simulink subsystem "HO_VectorBox"  (R2019b)
settings: Solver=VariableStepAuto  StartTime=0.0  StopTime=10.0  RelTol=1e-3
libraries: canmsglib x8, c280xlib x8, FunctionCallDivider x3
settings Model: Creator=Nick  LastModifiedBy=Nick

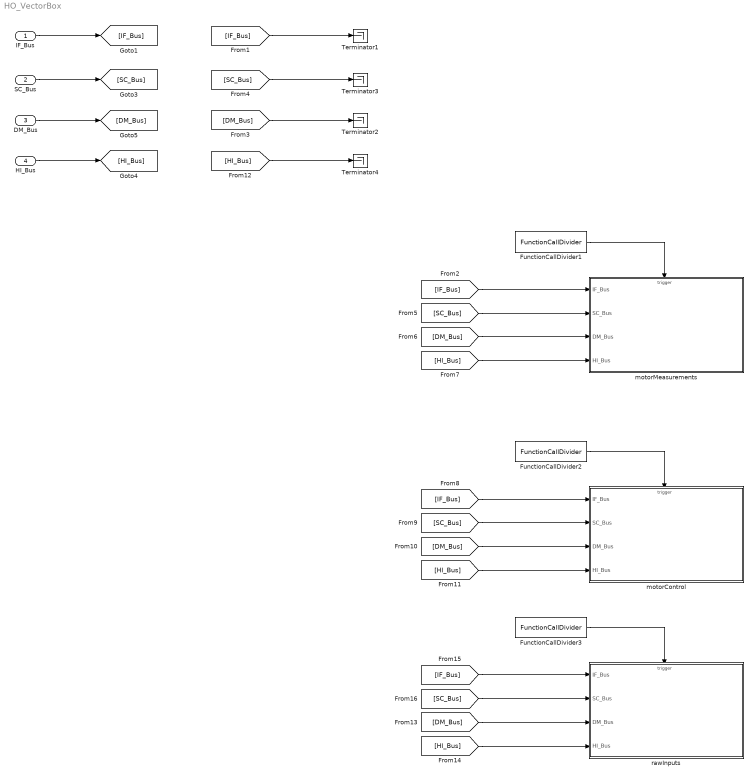
== system HO_VectorBox ==
  IF_Bus : Inport
  SC_Bus : Inport  Port=2
  DM_Bus : Inport  Port=3
  HI_Bus : Inport  Port=4
  FunctionCallDivider1 : FunctionCallDivider/Algroithms/FunctionCallDivider  counts=10
  FunctionCallDivider2 : FunctionCallDivider/Algroithms/FunctionCallDivider  counts=1
  FunctionCallDivider3 : FunctionCallDivider/Algroithms/FunctionCallDivider  counts=10
  Terminator{1..4} (4 alike) : Terminator
  motorControl : Subsystem  TreatAsAtomicUnit=on
  motorMeasurements : Subsystem  TreatAsAtomicUnit=on
  rawInputs : Subsystem  TreatAsAtomicUnit=on
  wires:
  [IF_Bus] -> motorMeasurements/1(IF_Bus)
  FunctionCallDivider1/1 -> motorMeasurements/Trigger
  [SC_Bus] -> motorMeasurements/2(SC_Bus)
  [DM_Bus] -> motorMeasurements/3(DM_Bus)
  [HI_Bus] -> motorMeasurements/4(HI_Bus)
  [HI_Bus] -> motorControl/4(HI_Bus)
  [DM_Bus] -> motorControl/3(DM_Bus)
  [IF_Bus] -> motorControl/1(IF_Bus)
  FunctionCallDivider2/1 -> motorControl/Trigger
  [SC_Bus] -> motorControl/2(SC_Bus)
  [IF_Bus] -> Terminator1/1
  [DM_Bus] -> Terminator2/1
  [SC_Bus] -> Terminator3/1
  DM_Bus/1 -> [DM_Bus]
  SC_Bus/1 -> [SC_Bus]
  HI_Bus/1 -> [HI_Bus]
  [HI_Bus] -> Terminator4/1
  IF_Bus/1 -> [IF_Bus]
  [SC_Bus] -> rawInputs/2(SC_Bus)
  [HI_Bus] -> rawInputs/4(HI_Bus)
  FunctionCallDivider3/1 -> rawInputs/Trigger
  [DM_Bus] -> rawInputs/3(DM_Bus)
  [IF_Bus] -> rawInputs/1(IF_Bus)

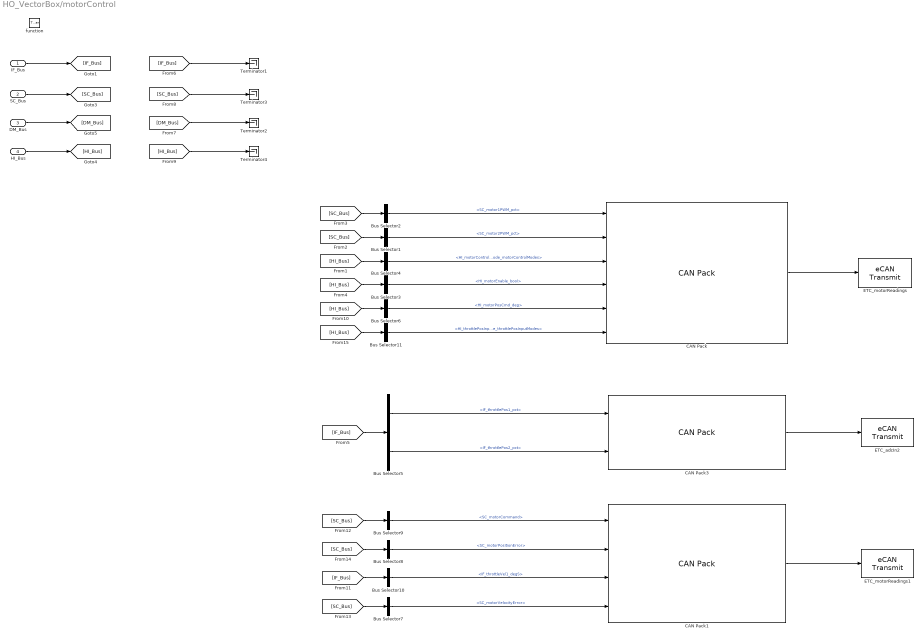
== system HO_VectorBox/motorControl ==
  IF_Bus : Inport
  SC_Bus : Inport  Port=2
  DM_Bus : Inport  Port=3
  HI_Bus : Inport  Port=4
  function : TriggerPort  TriggerType=function-call  VariantControl=Variant
  Bus Selector1 : BusSelector  OutputSignals=motorControlBus.SC_motor2PWM_pct
  Bus Selector10 : BusSelector  OutputSignals=AnalogInputFiltering_Bus.ExternalADCBus.IF_throttleVel1_degS
  Bus Selector11 : BusSelector  OutputSignals=VectorBoxBus.HI_throttlePosInputMode_throttlePosInputModes
  Bus Selector2 : BusSelector  OutputSignals=motorControlBus.SC_motor1PWM_pct
  Bus Selector3 : BusSelector  OutputSignals=VectorBoxBus.HI_motorEnable_bool
  Bus Selector4 : BusSelector  OutputSignals=VectorBoxBus.HI_motorControlMode_motorControlModes
  Bus Selector5 : BusSelector  OutputSignals=AnalogInputFiltering_Bus.ExternalADCBus.IF_throttlePos1_pct,AnalogInputFiltering_Bus.ExternalADCBus.IF_throttlePos2_pct
  Bus Selector6 : BusSelector  OutputSignals=VectorBoxBus.HI_motorPosCmd_deg
  Bus Selector7 : BusSelector  OutputSignals=motorControlBus.SC_motorVelocityError
  Bus Selector8 : BusSelector  OutputSignals=motorControlBus.SC_motorPositionError
  Bus Selector9 : BusSelector  OutputSignals=motorControlBus.SC_motorCommand
  CAN Pack : canmsglib/CAN Pack  CANdbFile=C:\Git\ETC-Development\DBCs\etc_benchTest.dbc  MsgList=ETC_motorControl  MsgName=ETC_motorControl  MsgIDType=Standard (11-bit identifier)  MsgIdentifier=1001  MsgLength=6  Remote=off  ApplyMinMax=off  BusOutput=off  SignalInfo={'ETC_motor1PWM','0','8','LE','unsigned','Standard','0','1','0','0','255';'ETC_motor2PWM','8','8','LE','unsigned','Standard','0','1','0','0','255';'ETC_motorControlMode','16','8','LE','unsigned','Standard','0','1','0','0','255';'ETC_motorEnable','40','1','LE','unsigned','Standard','0','1','0','0','1';'ETC_motorPositionCmd','24','8','LE','unsigned','Standard','0','1','0','0','255';'ETC_throttlePosInputMode','32','8','LE','unsigned','Standard','0','1','0','0','255'}
      settings: SourceProductName=Vehicle Network Toolbox  SourceProductBaseCode=VN  DataFormat=CANdb specified signals
  CAN Pack1 : canmsglib/CAN Pack  CANdbFile=C:\Git\ETC-Development\DBCs\etc_benchTest.dbc  MsgList=ETC_motorControlData1  MsgName=ETC_motorControlData1  MsgIDType=Standard (11-bit identifier)  MsgIdentifier=1002  MsgLength=8  Remote=off  ApplyMinMax=off  BusOutput=off  SignalInfo={'ETC_motorCommand','48','16','LE','signed','Standard','0','1','0','-32768','32767';'ETC_motorPositionError','0','16','LE','signed','Standard','0','0.01','0','-327.68','327.67';'ETC_motorVelocity','16','16','LE','signed','Standard','0','0.01','0','-327.68','327.67';'ETC_motorVelocityError','32','16','LE','signed','Standard','0','0.01','0','-327.68','327.67'}
      settings: SourceProductName=Vehicle Network Toolbox  SourceProductBaseCode=VN  DataFormat=CANdb specified signals
  CAN Pack3 : canmsglib/CAN Pack  CANdbFile=C:\Git\ETC-Development\DBCs\etc_benchTest.dbc  MsgList=ETC_throttlePosition  MsgName=ETC_throttlePosition  MsgIDType=Standard (11-bit identifier)  MsgIdentifier=1010  MsgLength=4  Remote=off  ApplyMinMax=off  BusOutput=off  SignalInfo={'ETC_throttlePosition1','0','16','LE','unsigned','Standard','0','0.01','0','0','655.35';'ETC_throttlePosition2','16','16','LE','unsigned','Standard','0','0.01','0','0','655.35'}
      settings: SourceProductName=Vehicle Network Toolbox  SourceProductBaseCode=VN  DataFormat=CANdb specified signals
  ETC_adcIn2 : c280xlib/eCAN Transmit  chipFamily=C280x  useModule=eCAN_A  mailboxNo=7  messageID=0  messageType=Standard (11-bit identifier)  enableBlockingMode=off  postInterrupt=off  interruptLine=0
      settings: SourceProductName=Embedded Coder Support Package for Texas Instruments C2000 Processors  SourceProductBaseCode=TIC2000
  ETC_motorReadings : c280xlib/eCAN Transmit  chipFamily=C280x  useModule=eCAN_A  mailboxNo=4  messageID=0  messageType=Standard (11-bit identifier)  enableBlockingMode=off  postInterrupt=off  interruptLine=0
      settings: SourceProductName=Embedded Coder Support Package for Texas Instruments C2000 Processors  SourceProductBaseCode=TIC2000
  ETC_motorReadings1 : c280xlib/eCAN Transmit  chipFamily=C280x  useModule=eCAN_A  mailboxNo=10  messageID=0  messageType=Standard (11-bit identifier)  enableBlockingMode=off  postInterrupt=off  interruptLine=0
      settings: SourceProductName=Embedded Coder Support Package for Texas Instruments C2000 Processors  SourceProductBaseCode=TIC2000
  Terminator{1..4} (4 alike) : Terminator
  wires:
  [HI_Bus] -> Bus Selector11/1
  Bus Selector11/1 -> CAN Pack/6  "<HI_throttlePosInputMode_throttlePosInputModes>"
  [SC_Bus] -> Bus Selector9/1
  Bus Selector9/1 -> CAN Pack1/1  "<SC_motorCommand>"
  [SC_Bus] -> Bus Selector7/1
  Bus Selector8/1 -> CAN Pack1/2  "<SC_motorPositionError>"
  Bus Selector10/1 -> CAN Pack1/3  "<IF_throttleVel1_degS>"
  [IF_Bus] -> Bus Selector10/1
  [SC_Bus] -> Bus Selector8/1
  CAN Pack1/1 -> ETC_motorReadings1/1
  Bus Selector7/1 -> CAN Pack1/4  "<SC_motorVelocityError>"
  IF_Bus/1 -> [IF_Bus]
  [HI_Bus] -> Terminator4/1
  HI_Bus/1 -> [HI_Bus]
  SC_Bus/1 -> [SC_Bus]
  DM_Bus/1 -> [DM_Bus]
  [SC_Bus] -> Terminator3/1
  [DM_Bus] -> Terminator2/1
  [IF_Bus] -> Terminator1/1
  Bus Selector5/1 -> CAN Pack3/1  "<IF_throttlePos1_pct>"
  CAN Pack3/1 -> ETC_adcIn2/1
  [IF_Bus] -> Bus Selector5/1
  Bus Selector5/2 -> CAN Pack3/2  "<IF_throttlePos2_pct>"
  Bus Selector3/1 -> CAN Pack/4  "<HI_motorEnable_bool>"
  Bus Selector1/1 -> CAN Pack/2  "<SC_motor2PWM_pct>"
  Bus Selector2/1 -> CAN Pack/1  "<SC_motor1PWM_pct>"
  [SC_Bus] -> Bus Selector1/1
  [HI_Bus] -> Bus Selector3/1
  [SC_Bus] -> Bus Selector2/1
  CAN Pack/1 -> ETC_motorReadings/1
  Bus Selector4/1 -> CAN Pack/3  "<HI_motorControlMode_motorControlModes>"
  [HI_Bus] -> Bus Selector4/1
  Bus Selector6/1 -> CAN Pack/5  "<HI_motorPosCmd_deg>"
  [HI_Bus] -> Bus Selector6/1

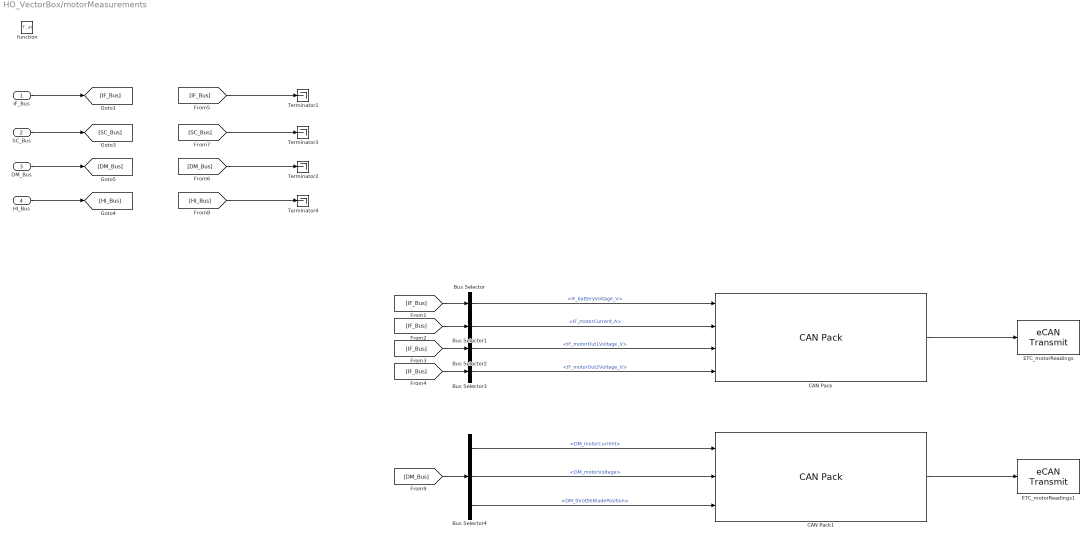
== system HO_VectorBox/motorMeasurements ==
  IF_Bus : Inport
  SC_Bus : Inport  Port=2
  DM_Bus : Inport  Port=3
  HI_Bus : Inport  Port=4
  function : TriggerPort  TriggerType=function-call  VariantControl=Variant
  Bus Selector : BusSelector  OutputSignals=AnalogInputFiltering_Bus.OnboardADCBus.IF_batteryVoltage_V
  Bus Selector1 : BusSelector  OutputSignals=AnalogInputFiltering_Bus.OnboardADCBus.IF_motorCurrent_A
  Bus Selector2 : BusSelector  OutputSignals=AnalogInputFiltering_Bus.OnboardADCBus.IF_motorOut1Voltage_V
  Bus Selector3 : BusSelector  OutputSignals=AnalogInputFiltering_Bus.OnboardADCBus.IF_motorOut2Voltage_V
  Bus Selector4 : BusSelector  OutputSignals=ETBModel_Bus.DM_motorCurrent,ETBModel_Bus.DM_motorVoltage,ETBModel_Bus.DM_throttleBladePosition
  CAN Pack : canmsglib/CAN Pack  CANdbFile=C:\Git\ETC-Development\DBCs\etc_benchTest.dbc  MsgList=ETC_motorMeasurements  MsgName=ETC_motorMeasurements  MsgIDType=Standard (11-bit identifier)  MsgIdentifier=1000  MsgLength=8  Remote=off  ApplyMinMax=off  BusOutput=off  SignalInfo={ 'ETC_batteryVoltage', '16', '16', 'LE', 'signed', 'Standard', '0', '0.001', '0', '-32.768', '32.767'; 'ETC_motorCurrent', '0', '16', 'LE', 'signed', 'Standard', '0', '0.001', '0', '-32.768', '32.767'; 'ETC_motorOut1Voltage', '32', '16', 'LE', 'signed', 'Standard', '0', '0.001', '0', '-32.768', '32.767'; 'ETC_motorOut2Voltage', '48', '16', 'LE', 'signed', 'Standard', '0', '0.001', '0', '-32.768', '32.767' }
      settings: SourceProductName=Vehicle Network Toolbox  SourceProductBaseCode=VN  DataFormat=CANdb specified signals
  CAN Pack1 : canmsglib/CAN Pack  CANdbFile=C:\Git\ETC-Development\DBCs\etc_benchTest.dbc  MsgList=ETC_modelOutput1  MsgName=ETC_modelOutput1  MsgIDType=Standard (11-bit identifier)  MsgIdentifier=1030  MsgLength=6  Remote=off  ApplyMinMax=off  BusOutput=off  SignalInfo={'ETC_modelMotorCurrent','16','16','LE','signed','Standard','0','0.001','0','-32.768','32.767';'ETC_modelMotorVoltage','32','16','LE','signed','Standard','0','0.001','0','-32.768','32.767';'ETC_modelThrottleBladePosition','0','8','LE','unsigned','Standard','0','0.01','0','0','2.55'}
      settings: SourceProductName=Vehicle Network Toolbox  SourceProductBaseCode=VN  DataFormat=CANdb specified signals
  ETC_motorReadings : c280xlib/eCAN Transmit  chipFamily=C280x  useModule=eCAN_A  mailboxNo=3  messageID=0  messageType=Standard (11-bit identifier)  enableBlockingMode=off  postInterrupt=off  interruptLine=0
      settings: SourceProductName=Embedded Coder Support Package for Texas Instruments C2000 Processors  SourceProductBaseCode=TIC2000
  ETC_motorReadings1 : c280xlib/eCAN Transmit  chipFamily=C280x  useModule=eCAN_A  mailboxNo=8  messageID=0  messageType=Standard (11-bit identifier)  enableBlockingMode=off  postInterrupt=off  interruptLine=0
      settings: SourceProductName=Embedded Coder Support Package for Texas Instruments C2000 Processors  SourceProductBaseCode=TIC2000
  Terminator{1..4} (4 alike) : Terminator
  wires:
  IF_Bus/1 -> [IF_Bus]
  [HI_Bus] -> Terminator4/1
  HI_Bus/1 -> [HI_Bus]
  SC_Bus/1 -> [SC_Bus]
  DM_Bus/1 -> [DM_Bus]
  [SC_Bus] -> Terminator3/1
  [DM_Bus] -> Terminator2/1
  [IF_Bus] -> Terminator1/1
  CAN Pack/1 -> ETC_motorReadings/1
  [IF_Bus] -> Bus Selector/1
  [IF_Bus] -> Bus Selector1/1
  [IF_Bus] -> Bus Selector2/1
  [IF_Bus] -> Bus Selector3/1
  Bus Selector3/1 -> CAN Pack/4  "<IF_motorOut2Voltage_V>"
  Bus Selector2/1 -> CAN Pack/3  "<IF_motorOut1Voltage_V>"
  Bus Selector1/1 -> CAN Pack/2  "<IF_motorCurrent_A>"
  Bus Selector/1 -> CAN Pack/1  "<IF_batteryVoltage_V>"
  Bus Selector4/1 -> CAN Pack1/1  "<DM_motorCurrent>"
  CAN Pack1/1 -> ETC_motorReadings1/1
  [DM_Bus] -> Bus Selector4/1
  Bus Selector4/3 -> CAN Pack1/3  "<DM_throttleBladePosition>"
  Bus Selector4/2 -> CAN Pack1/2  "<DM_motorVoltage>"

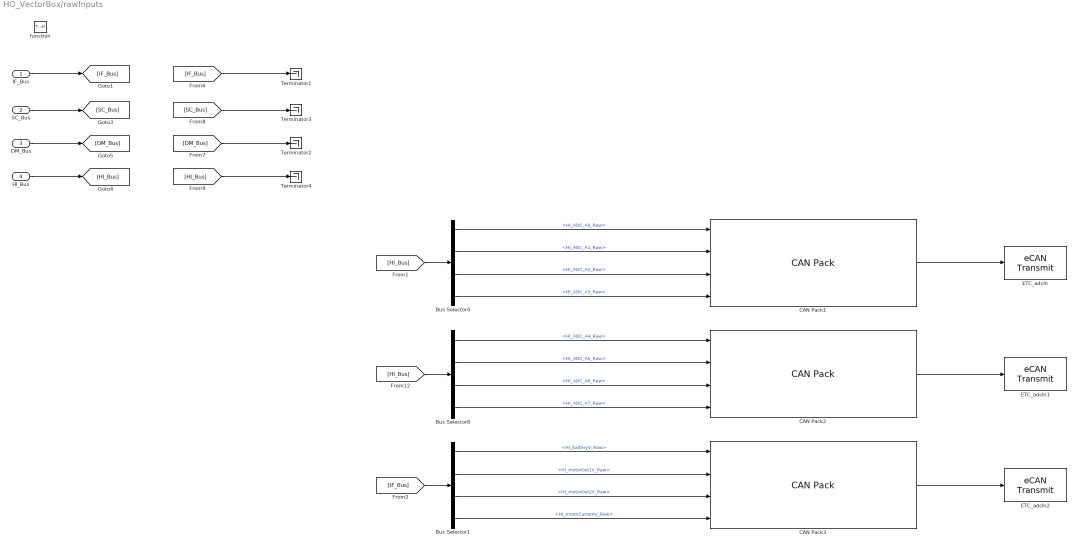
== system HO_VectorBox/rawInputs ==
  IF_Bus : Inport
  SC_Bus : Inport  Port=2
  DM_Bus : Inport  Port=3
  HI_Bus : Inport  Port=4
  function : TriggerPort  TriggerType=function-call  VariantControl=Variant
  Bus Selector1 : BusSelector  OutputSignals=AnalogInputFiltering_Bus.OnboardADCBus.HI_batteryV_Raw,AnalogInputFiltering_Bus.OnboardADCBus.HI_motorOut1V_Raw,AnalogInputFiltering_Bus.OnboardADCBus.HI_motorOut2V_Raw,AnalogInputFiltering_Bus.OnboardADCBus.HI_motorCurrentV_Raw
  Bus Selector4 : BusSelector  OutputSignals=SPIBus.HI_ADC_A0_Raw,SPIBus.HI_ADC_A1_Raw,SPIBus.HI_ADC_A2_Raw,SPIBus.HI_ADC_A3_Raw
  Bus Selector8 : BusSelector  OutputSignals=SPIBus.HI_ADC_A4_Raw,SPIBus.HI_ADC_A5_Raw,SPIBus.HI_ADC_A6_Raw,SPIBus.HI_ADC_A7_Raw
  CAN Pack1 : canmsglib/CAN Pack  CANdbFile=C:\Git\ETC-Development\DBCs\etc_benchTest.dbc  MsgList=ETC_adcRaw1  MsgName=ETC_adcRaw1  MsgIDType=Standard (11-bit identifier)  MsgIdentifier=1020  MsgLength=8  Remote=off  ApplyMinMax=off  BusOutput=off  SignalInfo={'ETC_extADC_A0_Raw','0','16','LE','unsigned','Standard','0','1','0','-Inf','Inf';'ETC_extADC_A1_Raw','16','16','LE','unsigned','Standard','0','1','0','-Inf','Inf';'ETC_extADC_A2_Raw','32','16','LE','unsigned','Standard','0','1','0','-Inf','Inf';'ETC_extADC_A3_Raw','48','16','LE','unsigned','Standard','0','1','0','-Inf','Inf'}
      settings: SourceProductName=Vehicle Network Toolbox  SourceProductBaseCode=VN  DataFormat=CANdb specified signals
  CAN Pack2 : canmsglib/CAN Pack  CANdbFile=C:\Git\ETC-Development\DBCs\etc_benchTest.dbc  MsgList=ETC_adcRaw2  MsgName=ETC_adcRaw2  MsgIDType=Standard (11-bit identifier)  MsgIdentifier=1021  MsgLength=8  Remote=off  ApplyMinMax=off  BusOutput=off  SignalInfo={'ETC_extADC_A4_Raw','0','16','LE','unsigned','Standard','0','1','0','-Inf','Inf';'ETC_extADC_A5_Raw','16','16','LE','unsigned','Standard','0','1','0','-Inf','Inf';'ETC_extADC_A6_Raw','32','16','LE','unsigned','Standard','0','1','0','-Inf','Inf';'ETC_extADC_A7_Raw','48','16','LE','unsigned','Standard','0','1','0','-Inf','Inf'}
      settings: SourceProductName=Vehicle Network Toolbox  SourceProductBaseCode=VN  DataFormat=CANdb specified signals
  CAN Pack3 : canmsglib/CAN Pack  CANdbFile=C:\Git\ETC-Development\DBCs\etc_benchTest.dbc  MsgList=ETC_adcRaw3  MsgName=ETC_adcRaw3  MsgIDType=Standard (11-bit identifier)  MsgIdentifier=1022  MsgLength=8  Remote=off  ApplyMinMax=off  BusOutput=off  SignalInfo={'ETC_c2000ADC_batteryVoltage_Raw','16','16','LE','unsigned','Standard','0','1','0','-Inf','Inf';'ETC_c2000ADC_motor1voltage_Raw','32','16','LE','unsigned','Standard','0','1','0','-Inf','Inf';'ETC_c2000ADC_motor2voltage_Raw','48','16','LE','unsigned','Standard','0','1','0','-Inf','Inf';'ETC_c2000ADC_motorCurrent_Raw','0','16','LE','unsigned','Standard','0','1','0','-Inf','Inf'}
      settings: SourceProductName=Vehicle Network Toolbox  SourceProductBaseCode=VN  DataFormat=CANdb specified signals
  ETC_adcIn : c280xlib/eCAN Transmit  chipFamily=C280x  useModule=eCAN_A  mailboxNo=5  messageID=0  messageType=Standard (11-bit identifier)  enableBlockingMode=off  postInterrupt=off  interruptLine=0
      settings: SourceProductName=Embedded Coder Support Package for Texas Instruments C2000 Processors  SourceProductBaseCode=TIC2000
  ETC_adcIn1 : c280xlib/eCAN Transmit  chipFamily=C280x  useModule=eCAN_A  mailboxNo=6  messageID=0  messageType=Standard (11-bit identifier)  enableBlockingMode=off  postInterrupt=off  interruptLine=0
      settings: SourceProductName=Embedded Coder Support Package for Texas Instruments C2000 Processors  SourceProductBaseCode=TIC2000
  ETC_adcIn2 : c280xlib/eCAN Transmit  chipFamily=C280x  useModule=eCAN_A  mailboxNo=9  messageID=0  messageType=Standard (11-bit identifier)  enableBlockingMode=off  postInterrupt=off  interruptLine=0
      settings: SourceProductName=Embedded Coder Support Package for Texas Instruments C2000 Processors  SourceProductBaseCode=TIC2000
  Terminator{1..4} (4 alike) : Terminator
  wires:
  [IF_Bus] -> Bus Selector1/1
  Bus Selector1/3 -> CAN Pack3/3  "<HI_motorOut2V_Raw>"
  CAN Pack3/1 -> ETC_adcIn2/1
  Bus Selector1/2 -> CAN Pack3/2  "<HI_motorOut1V_Raw>"
  Bus Selector1/1 -> CAN Pack3/1  "<HI_batteryV_Raw>"
  Bus Selector1/4 -> CAN Pack3/4  "<HI_motorCurrentV_Raw>"
  IF_Bus/1 -> [IF_Bus]
  [HI_Bus] -> Terminator4/1
  HI_Bus/1 -> [HI_Bus]
  SC_Bus/1 -> [SC_Bus]
  DM_Bus/1 -> [DM_Bus]
  [SC_Bus] -> Terminator3/1
  [DM_Bus] -> Terminator2/1
  [IF_Bus] -> Terminator1/1
  Bus Selector4/2 -> CAN Pack1/2  "<HI_ADC_A1_Raw>"
  Bus Selector4/3 -> CAN Pack1/3  "<HI_ADC_A2_Raw>"
  Bus Selector4/4 -> CAN Pack1/4  "<HI_ADC_A3_Raw>"
  Bus Selector8/2 -> CAN Pack2/2  "<HI_ADC_A5_Raw>"
  Bus Selector8/3 -> CAN Pack2/3  "<HI_ADC_A6_Raw>"
  Bus Selector8/4 -> CAN Pack2/4  "<HI_ADC_A7_Raw>"
  [HI_Bus] -> Bus Selector8/1
  CAN Pack2/1 -> ETC_adcIn1/1
  Bus Selector8/1 -> CAN Pack2/1  "<HI_ADC_A4_Raw>"
  CAN Pack1/1 -> ETC_adcIn/1
  [HI_Bus] -> Bus Selector4/1
  Bus Selector4/1 -> CAN Pack1/1  "<HI_ADC_A0_Raw>"
